simulink model "controller_testing_FILTERED"  (R2023b)
settings: Solver=VariableStepAuto  StartTime=0.0  StopTime=100  RelTol=1e-3
values from neighbouring files (symbols this model uses):
  tvs =     [tvs_parameters.mat]
settings Model: Creator=Inver  LastModifiedBy=Inver
settings OptimizationCC: DefaultParameterBehavior=Inlined  UseDivisionForNetSlopeComputation=on  GainParamInheritBuiltInType=on  UseFloatMulNetSlope=on  InlineInvariantSignals=on  PassReuseOutputArgsAs=Individual arguments  ZeroExternalMemoryAtStartup=off  ZeroInternalMemoryAtStartup=off  NoFixptDivByZeroProtection=on  EfficientFloat2IntCast=on  LifeSpan=1  OptimizeBlockOrder=speed  OptimizationPriority=Speed  MultiThreadedLoops=on  EfficientTunableParamExpr=on
settings DebuggingCC: ParameterTunabilityLossMsg=error
settings HardwareCC: ProdBitPerPointer=32  ProdBitPerSizeT=32  ProdBitPerPtrDiffT=32  ProdLargestAtomicInteger=Long  ProdLargestAtomicFloat=Double  ProdWordSize=32  ProdLongLongMode=on  ProdHWDeviceType=ARM Compatible->ARM Cortex-M
settings SFSimCC: SimCustomHeaderCode="#include \"simplex.h\""  SimUserSources=simplex.c  MATLABDynamicMemAlloc=off
settings RTWCC: Description=Embedded Coder  SystemTargetFile=ert.tlc  GenCodeOnly=on  PackageGeneratedCodeAndArtifacts=on  TemplateMakefile=ert_default_tmf  Toolchain=GNU Tools for ARM Embedded Processors  BuildConfiguration=Faster Runs  CodeExecutionProfiling=on  CodeProfilingInstrumentation=detailed
settings CodeAppCC: ForceParamTrailComments=on  IgnoreCustomStorageClasses=off  OperatorAnnotations=on  SimulinkDataObjDesc=on  SFDataObjDesc=on  CustomSymbolStrGlobalVar=rt$N$M  CustomSymbolStrType=$N$M  CustomSymbolStrFcn=$N$M$F  CustomSymbolStrMacro=$N$M  InsertBlockDesc=on
settings ERTTargetCC: TargetLangStandard=C99 (ISO)  GenerateSampleERTMain=on  IncludeMdlTerminateFcn=off  CombineSignalStateStructs=on  CodeInterfacePackaging=Reusable function  SupportComplex=off  SupportNonInlinedSFcns=on  InlinedParameterPlacement=NonHierarchical  RootIOFormat=Structure reference  ERTCustomFileTemplate=example_file_process.tlc  GlobalDataDefinition=InSeparateSourceFile  DataDefinitionFile=data.c  GlobalDataReference=InSeparateHeaderFile  ERTFilePackagingFormat=CompactWithDataFile  DataReferenceFile=data.h

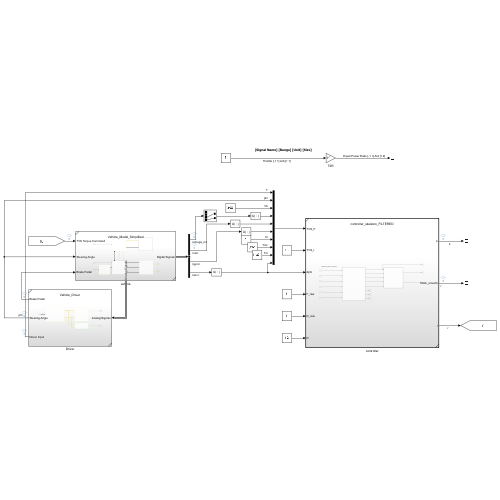
[thumbnail: Simulink's stored preview of the top-level diagram]
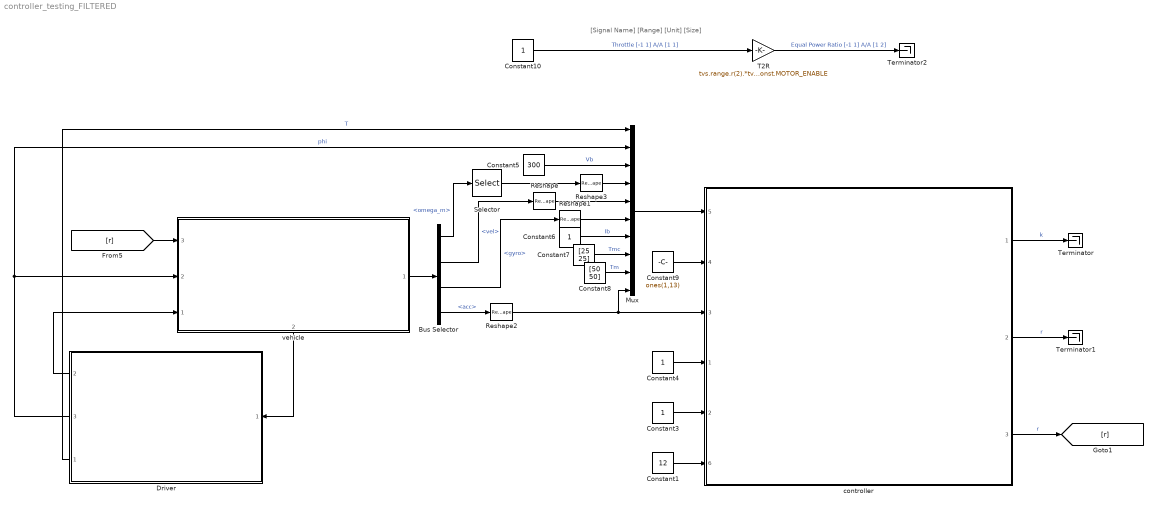
== system controller_testing_FILTERED ==
  note: [Signal Name] [Range] [Unit] [Size]
  Bus Selector : BusSelector  OutputSignals=Corner Dynamics Sensors.omega_m,Navigation Sensors.vel,Navigation Sensors.gyro,Navigation Sensors.acc
  Constant1 : Constant  Value=12
  Constant{3..4,6,10} (4 alike) : Constant
  Constant5 : Constant  Value=300
  Constant7 : Constant  Value=[25 25]
  Constant8 : Constant  Value=[50 50]
  Constant9 : Constant  Value=ones(1,13)  OutDataTypeStr=boolean
  Driver : Subsystem  ReferencedSubsystem=Vehicle_Driver
      settings: PortSchema="{\"entries\":[{\"content\":{\"sides\":[{\"content\":{\"connectorIds\":[\"Out2\",\"Out3\",\"Out1\"]},\"type\":\"ConnectorPlacement.EquallySpacedRectSide\",\"uuid\":\"c8f3518c-48c1-48e6-bf49-b5946aebc156\"},{\"content\":{\"connectorIds\":[\"In1\"],\"side\":\"RIGHT\"},\"type\":\"ConnectorPlacement.EquallySpacedRectSide\",\"uuid\":\"d1ff2ecd-3804-4616-be8b-c7741816ffed\"},{\"content\":{\"side\":\"TOP\"},\"type\":\"ConnectorPlacement.EquallySpacedRectSide\",\"uuid\":\"0d6b10aa-d497-4cfd-b6f3-3ffc80b2cc8c\"}]},\"type\":\"ConnectorPlacement.EquallySpacedConnector\",\"uuid\":\"8189dedf-d1b1-471b-a005-48bc7d1d6f32\"}],\"packageUris\":[\"http://schema.mathworks.com/mf0/Connector/R2020b\"],\"version\":\"1.0\"}"
  Mux : Mux  Inputs=10
  Reshape{,1..3} (4 alike) : Reshape
  Selector : Selector  InputPortWidth=4  IndexOptions=Index vector (dialog)  Indices=[3 4]  OutputSizes=1
  T2R : Gain  Gain=tvs.range.r(2).*tvs.const.MOTOR_ENABLE  OutDataTypeStr=double
  Terminator : Terminator
  Terminator1 : Terminator
  Terminator2 : Terminator
  controller : Subsystem  TreatAsAtomicUnit=on  SystemSampleTime=0.02  ReferencedSubsystem=controller_skeleton_FILTERED
      settings: PortSchema="{\"entries\":[{\"content\":{\"sides\":[{\"content\":{\"connectorIds\":[\"In5\",\"In4\",\"In3\",\"In1\",\"In2\",\"In6\"]},\"type\":\"ConnectorPlacement.EquallySpacedRectSide\",\"uuid\":\"52b1df42-6e7f-45d3-b7c9-232c4418f487\"},{\"content\":{\"connectorIds\":[\"Out1\",\"Out2\",\"Out3\"],\"side\":\"RIGHT\"},\"type\":\"ConnectorPlacement.EquallySpacedRectSide\",\"uuid\":\"e4c52b5d-e43f-4131-af39-863e21bd5493\"},{\"content\":{\"side\":\"TOP\"},\"type\":\"ConnectorPlacement.EquallySpacedRectSide\",\"uuid\":\"e8efffec-e2c6-4a68-bbcf-545da82a33a9\"}]},\"type\":\"ConnectorPlacement.EquallySpacedConnector\",\"uuid\":\"e642afc6-31fe-4ac7-95bb-2149c1d24da1\"}],\"packageUris\":[\"http://schema.mathworks.com/mf0/Connector/R2020b\"],\"version\":\"1.0\"}"
  vehicle : Subsystem  ReferencedSubsystem=Vehicle_Model_Simplified
      settings: PortSchema="{\"entries\":[{\"content\":{\"sides\":[{\"content\":{\"connectorIds\":[\"In3\",\"In2\",\"In1\"]},\"type\":\"ConnectorPlacement.EquallySpacedRectSide\",\"uuid\":\"8b7d0458-19e6-4f5f-a2ba-6896bc8547a5\"},{\"content\":{\"connectorIds\":[\"Out1\"],\"side\":\"RIGHT\"},\"type\":\"ConnectorPlacement.EquallySpacedRectSide\",\"uuid\":\"a43880ad-82fe-45ef-8c70-24ac571715de\"},{\"content\":{\"side\":\"TOP\"},\"type\":\"ConnectorPlacement.EquallySpacedRectSide\",\"uuid\":\"66574ddc-a488-4804-99cd-be4e95fcc69f\"},{\"content\":{\"connectorIds\":[\"Out2\"],\"side\":\"BOTTOM\"},\"type\":\"ConnectorPlacement.EquallySpacedRectSide\",\"uuid\":\"fabe72c8-70b5-4979-b7ad-47d1f12336ef\"}]},\"type\":\"ConnectorPlacement.EquallySpacedConnector\",\"uuid\":\"a0af0009-be5b-43ca-b50b-758f5d04f5dc\"}],\"packageUris\":[\"http://schema.mathworks.com/mf0/Connector/R2020b\"],\"version\":\"1.0\"}"
  wires:
  controller/1 -> Terminator/1  "k"
  Driver/1 -> Mux/1  "T"
  Driver/3 -> Mux/2, vehicle/2  "phi"
  Driver/2 -> vehicle/1
  vehicle/1 -> Bus Selector/1
  [r] -> vehicle/3
  vehicle/2 -> Driver/1
  controller/3 -> [r]  "r"
  Constant1/1 -> controller/6
  Constant3/1 -> controller/2
  Constant4/1 -> controller/1
  Constant5/1 -> Mux/3  "Vb"
  Bus Selector/1 -> Selector/1  "<omega_m>"
  Bus Selector/2 -> Reshape/1  "<vel>"
  Bus Selector/3 -> Reshape1/1  "<gyro>"
  Bus Selector/4 -> Reshape2/1  "<acc>"
  Constant6/1 -> Mux/7  "Ib"
  Constant7/1 -> Mux/8  "Tmc"
  Constant8/1 -> Mux/9  "Tm"
  Mux/1 -> controller/5
  Constant10/1 -> T2R/1  "Throttle [-1 1] A/A [1 1]"
  Constant9/1 -> controller/4
  controller/2 -> Terminator1/1  "r"
  T2R/1 -> Terminator2/1  "Equal Power Ratio [-1 1] A/A [1 2]"
  Reshape/1 -> Mux/5
  Reshape1/1 -> Mux/6
  Reshape3/1 -> Mux/4
  Selector/1 -> Reshape3/1
  Reshape2/1 -> Mux/10, controller/3
